simulink model "ame532Project1_GimbalDynamicsModel_2023a_Editing"  (R2023a)
settings: Solver=ode4  StartTime=0.0  StopTime=120  FixedStep=0.01  RelTol=1e-3
model workspace (MAT data in the model file):
  theta = Simulink.Parameter
  theta.DataType = 'auto'
  theta.Complexity = 'real'
  theta.Dimensions = [0 0]
values from neighbouring files (symbols this model uses):
  elevator_sA = 0.435    [Sim_sixDOFdriverScript.m]
  Jxx = 1    [Sim_sixDOFdriverScript.m]
  Jxy = 0.    (= 0)    [Sim_sixDOFdriverScript.m]
  Jxz = 3    [Sim_sixDOFdriverScript.m]
  Jyx = 2    [Sim_sixDOFdriverScript.m]
  Jyy = 2    [Sim_sixDOFdriverScript.m]
  Jyz = 0    [Sim_sixDOFdriverScript.m]
  Jzx = Jxz    (= 3)    [Sim_sixDOFdriverScript.m]
  Jzy = Jyz    (= 0)    [Sim_sixDOFdriverScript.m]
  Jzz = 2    [Sim_sixDOFdriverScript.m]
  leftaileron_sA = 0.192/2    (= 0.096)    [Sim_sixDOFdriverScript.m]
  LL = 0.8    [Sim_sixDOFdriverScript.m]
  MM = 0.8    [Sim_sixDOFdriverScript.m]
  NN = 0.8    [Sim_sixDOFdriverScript.m]
  rEarth = 6378100    [Sim_sixDOFdriverScript.m]
  rightaileron_sA = 0.192/2    (= 0.096)    [Sim_sixDOFdriverScript.m]
  rudder_sA = 0.0333    [Sim_sixDOFdriverScript.m]
  totMass = sum(componentMassesAndGeom(:,1))    [computeMassProps.m]
  x_S2_B_B = (x_S2_B_B_nominal + [0.25*c_s2 0 0]') - x_cg    [computeMassProps.m]
  x_S3_B_B = (x_S3_B_B_nominal + [0.25*c_s3 0 0]') - x_cg    [computeMassProps.m]
  x_S4_B_B = (x_S4_B_B_nominal + [0.25*c_s4 0 0]') - x_cg    [computeMassProps.m]
  x_S5_B_B = (x_S5_B_B_nominal + [0.25*c_s5 0 0]') - x_cg    [computeMassProps.m]
undefined symbols (not defined in the file or in its folder): a0_s2, a0_s3, a0_s4, a0_s5, AR_s2, AR_s3, AR_s4, AR_s5, area_s2, area_s3, area_s4, area_s5, c_s2, c_s3, c_s4, c_s5, CD0_s2, CD0_s3, CD0_s4, CD0_s5, CDa_s2, CDa_s3, CDa_s4, CDa_s5, CL0_s2, CL0_s3, CL0_s4, CL0_s5, CM0_s2, CM0_s3, CM0_s4, CM0_s5, CMa_s2, CMa_s3, CMa_s4, CMa_s5, e_s2, e_s3, e_s4, e_s5, earthRadius, i_s2, i_s3, i_s4, i_s5, n_s2, n_s3, n_s4, n_s5, ro
libraries: simulink_extras x37, matrix_library x26, aerolibutil x6, aerolibfltsims x4, simulink x4, vrlib x3, aerolibtransform2 x2, slpidlib x2, sharedutil x1
(part 1 of 5)
settings Model: Creator=enson  LastModifiedBy=fahee
settings ModelReferenceCC: EnableRefExpFcnMdlSchedulingChecks=on

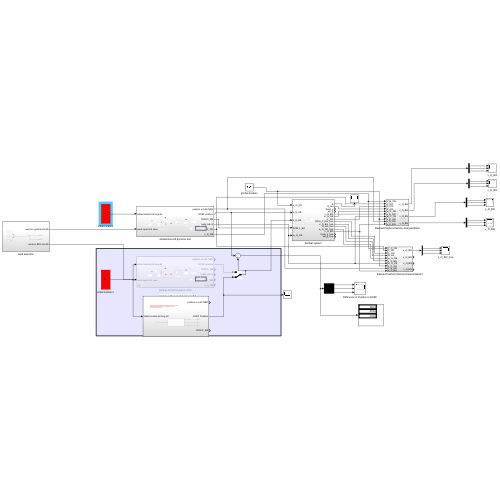
[thumbnail: Simulink's stored preview of the top-level diagram]
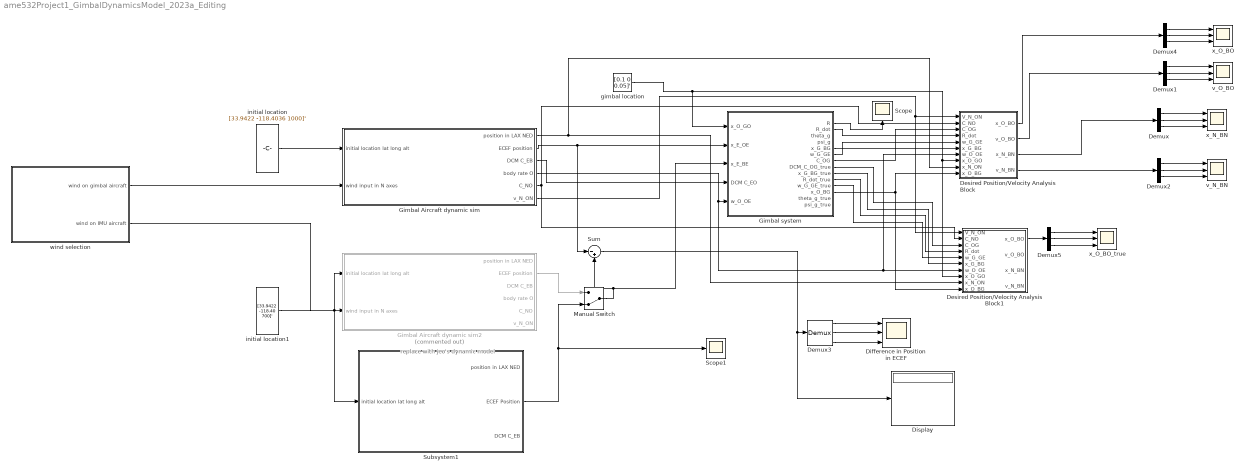
== system ame532Project1_GimbalDynamicsModel_2023a_Editing ==
  note: replace with jeo's dynamic model
  Demux{,1..5} (6 alike) : Demux  Outputs=3
  Desired Position/Velocity Analysis Block : Subsystem
  Desired Position/Velocity Analysis Block1 : Subsystem
  Difference in Position in ECEF : Scope  NumInputPorts=3
  Display : Display
  Gimbal Aircraft dynamic sim : Subsystem
  Gimbal Aircraft dynamic sim2 : Subsystem  Commented=on
  Gimbal system : Subsystem
  Manual Switch : ManualSwitch  CurrentSetting=0
  Scope : Scope
  Scope1 : Scope
  Subsystem1 : Subsystem
  Sum : Sum  Inputs=|-+
  gimbal location : Constant  Value=[0.1 0 0.05]'
  initial location : Constant  Value=[33.9422 -118.4036 1000]'
  initial location1 : Constant  Value=[33.9422 -118.40 700]'
  v_N_BN : Scope  NumInputPorts=3
  v_O_BO : Scope  NumInputPorts=3
  wind selection : Subsystem
  x_N_BN : Scope  NumInputPorts=3
  x_O_BO : Scope  NumInputPorts=3
  x_O_BO_true : Scope  NumInputPorts=3
  wires:
  gimbal location/1 -> Gimbal system/1(x_O_GO), Desired Position/Velocity Analysis Block1/8(x_O_GO), Desired Position/Velocity Analysis Block/8(x_O_GO)
  Gimbal Aircraft dynamic sim/2(ECEF position) -> Sum/1, Gimbal system/2(x_E_OE)
  Manual Switch/1 -> Sum/2, Gimbal system/3(x_E_BE)
  Gimbal system/1(R) -> Scope/1
  Gimbal Aircraft dynamic sim/3(DCM C_EB) -> Gimbal system/4(DCM C_EO)
  Demux3/3 -> Difference in Position in ECEF/3
  Demux3/2 -> Difference in Position in ECEF/2
  Demux3/1 -> Difference in Position in ECEF/1
  Sum/1 -> Display/1, Demux3/1
  initial location/1 -> Gimbal Aircraft dynamic sim/1(initial location lat long alt)
  initial location1/1 -> Subsystem1/1(initial location lat long alt), Gimbal Aircraft dynamic sim2/1(initial location lat long alt)
  Gimbal Aircraft dynamic sim/4(body rate O) -> Desired Position/Velocity Analysis Block/7(w_O_OE), Desired Position/Velocity Analysis Block1/7(w_O_OE), Gimbal system/5(w_O_OE)
  Gimbal system/7(C_OG) -> Desired Position/Velocity Analysis Block/3(C_OG)
  Gimbal system/5(x_G_BG) -> Desired Position/Velocity Analysis Block/6(x_G_BG)
  Gimbal Aircraft dynamic sim/1(position in LAX NED) -> Desired Position/Velocity Analysis Block1/9(x_N_ON), Desired Position/Velocity Analysis Block/9(x_N_ON)
  Gimbal system/2(R_dot) -> Desired Position/Velocity Analysis Block/4(R_dot)
  Gimbal system/6(w_G_GE) -> Desired Position/Velocity Analysis Block/5(w_G_GE)
  Gimbal Aircraft dynamic sim/5(C_NO) -> Desired Position/Velocity Analysis Block1/2(C_NO), Desired Position/Velocity Analysis Block/2(C_NO)
  Gimbal Aircraft dynamic sim/6(v_N_ON) -> Desired Position/Velocity Analysis Block1/1(V_N_ON), Desired Position/Velocity Analysis Block/1(V_N_ON)
  Desired Position/Velocity Analysis Block/3(x_N_BN) -> Demux/1
  Demux/1 -> x_N_BN/1
  Demux/2 -> x_N_BN/2
  Demux/3 -> x_N_BN/3
  Subsystem1/2(ECEF Position) -> Scope1/1, Manual Switch/2
  Gimbal Aircraft dynamic sim2/2(ECEF position) -> Manual Switch/1
  Gimbal system/9(x_G_BG_true) -> Desired Position/Velocity Analysis Block1/6(x_G_BG)
  Gimbal system/11(w_G_GE_true) -> Desired Position/Velocity Analysis Block1/5(w_G_GE)
  Gimbal system/10(R_dot_true) -> Desired Position/Velocity Analysis Block1/4(R_dot)
  Gimbal system/8(DCM_C_OG_true) -> Desired Position/Velocity Analysis Block1/3(C_OG)
  Gimbal system/12(x_O_BG) -> Desired Position/Velocity Analysis Block1/10(x_O_BG), Desired Position/Velocity Analysis Block/10(x_O_BG)
  Desired Position/Velocity Analysis Block/2(v_O_BO) -> Demux1/1
  Demux1/2 -> v_O_BO/2
  Demux1/1 -> v_O_BO/1
  Demux1/3 -> v_O_BO/3
  Desired Position/Velocity Analysis Block/4(v_N_BN) -> Demux2/1
  Demux2/2 -> v_N_BN/2
  Demux2/1 -> v_N_BN/1
  Demux2/3 -> v_N_BN/3
  Desired Position/Velocity Analysis Block/1(x_O_BO) -> Demux4/1
  Demux4/2 -> x_O_BO/2
  Demux4/1 -> x_O_BO/1
  Demux4/3 -> x_O_BO/3
  Desired Position/Velocity Analysis Block1/1(x_O_BO) -> Demux5/1
  Demux5/1 -> x_O_BO_true/1
  Demux5/3 -> x_O_BO_true/3
  Demux5/2 -> x_O_BO_true/2
  wind selection/1(wind on gimbal aircraft) -> Gimbal Aircraft dynamic sim/2(wind input in N axes)
  wind selection/2(wind on IMU aircraft) -> Gimbal Aircraft dynamic sim2/2(wind input in N axes)

== system ame532Project1_GimbalDynamicsModel_2023a_Editing/Desired Position//Velocity Analysis Block ==
  note: position of IMU aircraft w.r.t gimbal + position of gimbal w.r.t gimbal aircraft = position of IMU aircraft w.r.t gimbal aircraft in gimbal coordinates
  note: position of gimbal aircraft w.r.t NED in NED frame
  note: position of gimbal w.r.t aircraft in aircraft frame
  note: position of gimbal aircraft w.r.t Earth in gimbal aircraft frame
  note: Position of IMU aircraft w.r.t the Gimbal in Gimbal Frame
  note: gimbal rates w.r.t Earth in Gimbal frame
  note: derivative of distance from gimbal to IMU aircraft
  note: DCM gimbal to gimbal aircraft
  note: DCM gimbal aircraft to NED
  note: velocity of gimbal aircraft w.r.t NED
  V_N_ON : Inport
  C_NO : Inport  Port=2
  C_OG : Inport  Port=3
  R_dot : Inport  Port=4
  w_G_GE : Inport  Port=5
  x_G_BG : Inport  Port=6
  w_O_OE : Inport  Port=7
  x_O_GO : Inport  Port=8
  x_N_ON : Inport  Port=9
  x_O_BG : Inport  Port=10
  Constant : Constant  Value=0
  Constant1 : Constant  Value=0
  Cross Product : matrix_library/Cross Product
  Cross Product1 : matrix_library/Cross Product
  Display{,1..3,5..6} (6 alike) : Display
  Matrix Multiply{,1..8} (9 alike) : Product  Multiplication=Matrix(*)
  Mux : Mux  Inputs=3
  Scope : Scope
  Scope1 : Scope
  Scope2 : Scope
  Sum : Sum  Inputs=|++
  Sum1 : Sum  Inputs=|++
  Sum2 : Sum  Inputs=|+++
  Sum3 : Sum  Inputs=|++
  Sum4 : Sum  Inputs=|+++
  x_O_BO : Outport
  v_O_BO : Outport  Port=2
  x_N_BN : Outport  Port=3
  v_N_BN : Outport  Port=4
  wires:
  x_O_GO/1 -> Matrix Multiply3/2, Sum/1
  C_OG/1 -> Matrix Multiply5/1, Matrix Multiply2/1, Matrix Multiply1/1, Display5/1, Matrix Multiply/1
  x_G_BG/1 -> Matrix Multiply/2, Matrix Multiply2/2
  Matrix Multiply/1 -> Display3/1, Sum/2
  Sum/1 -> Matrix Multiply7/2, x_O_BO/1
  Constant/1 -> Mux/2
  Constant1/1 -> Mux/3
  R_dot/1 -> Mux/1
  Mux/1 -> Matrix Multiply1/2
  Matrix Multiply1/1 -> Sum3/1, Sum1/1
  Matrix Multiply2/1 -> Cross Product/2
  Cross Product/1 -> Sum1/2, Sum3/2
  Sum1/1 -> v_O_BO/1
  x_N_ON/1 -> Display2/1, Sum2/1, Scope2/1
  C_NO/1 -> Matrix Multiply8/1, Matrix Multiply7/1, Matrix Multiply6/1, Display6/1, Matrix Multiply4/1, Matrix Multiply3/1
  Matrix Multiply3/1 -> Display1/1, Scope/1, Sum2/2
  Matrix Multiply4/1 -> Display/1, Scope1/1, Sum2/3
  Sum2/1 -> x_N_BN/1
  Sum3/1 -> Matrix Multiply6/2
  Matrix Multiply7/1 -> Cross Product1/2
  Matrix Multiply8/1 -> Cross Product1/1
  w_O_OE/1 -> Matrix Multiply8/2
  Cross Product1/1 -> Sum4/3
  Sum4/1 -> v_N_BN/1
  Matrix Multiply6/1 -> Sum4/1
  V_N_ON/1 -> Sum4/2
  x_O_BG/1 -> Matrix Multiply4/2
  w_G_GE/1 -> Matrix Multiply5/2
  Matrix Multiply5/1 -> Cross Product/1

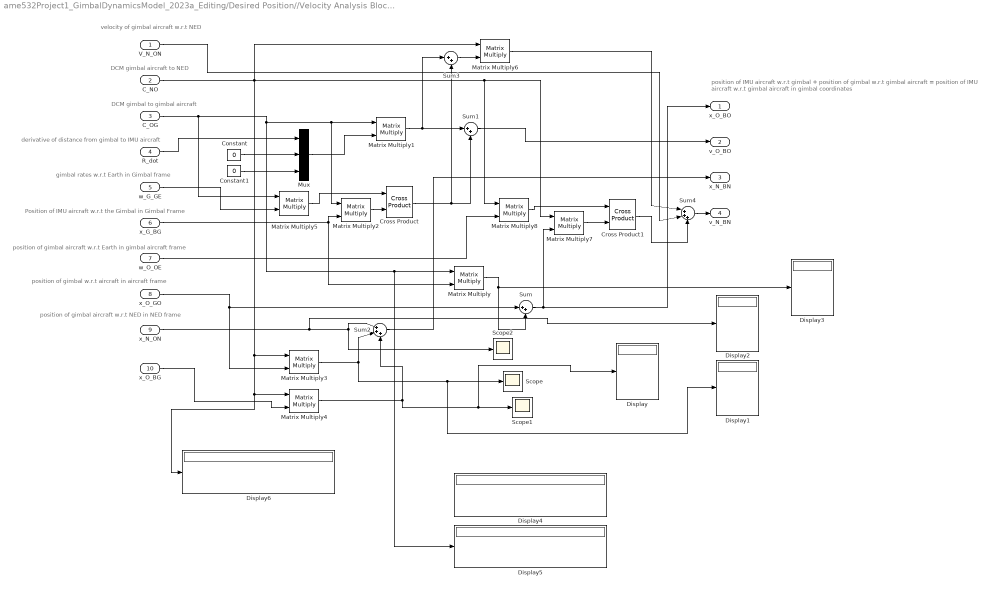
== system ame532Project1_GimbalDynamicsModel_2023a_Editing/Desired Position//Velocity Analysis Block1 ==
  note: position of IMU aircraft w.r.t gimbal + position of gimbal w.r.t gimbal aircraft = position of IMU aircraft w.r.t gimbal aircraft in gimbal coordinates
  note: position of gimbal aircraft w.r.t NED in NED frame
  note: position of gimbal w.r.t aircraft in aircraft frame
  note: position of gimbal aircraft w.r.t Earth in gimbal aircraft frame
  note: Position of IMU aircraft w.r.t the Gimbal in Gimbal Frame
  note: gimbal rates w.r.t Earth in Gimbal frame
  note: derivative of distance from gimbal to IMU aircraft
  note: DCM gimbal to gimbal aircraft
  note: DCM gimbal aircraft to NED
  note: velocity of gimbal aircraft w.r.t NED
  V_N_ON : Inport
  C_NO : Inport  Port=2
  C_OG : Inport  Port=3
  R_dot : Inport  Port=4
  w_G_GE : Inport  Port=5
  x_G_BG : Inport  Port=6
  w_O_OE : Inport  Port=7
  x_O_GO : Inport  Port=8
  x_N_ON : Inport  Port=9
  x_O_BG : Inport  Port=10
  Constant : Constant  Value=0
  Constant1 : Constant  Value=0
  Cross Product : matrix_library/Cross Product
  Cross Product1 : matrix_library/Cross Product
  Display{,1..6} (7 alike) : Display
  Matrix Multiply{,1..8} (9 alike) : Product  Multiplication=Matrix(*)
  Mux : Mux  Inputs=3
  Scope : Scope
  Scope1 : Scope
  Scope2 : Scope
  Sum : Sum  Inputs=|++
  Sum1 : Sum  Inputs=|++
  Sum2 : Sum  Inputs=|+++
  Sum3 : Sum  Inputs=|++
  Sum4 : Sum  Inputs=|+++
  x_O_BO : Outport
  v_O_BO : Outport  Port=2
  x_N_BN : Outport  Port=3
  v_N_BN : Outport  Port=4
  wires:
  x_O_GO/1 -> Matrix Multiply3/2, Sum/1
  C_OG/1 -> Matrix Multiply5/1, Matrix Multiply2/1, Matrix Multiply1/1, Display5/1, Matrix Multiply/1
  x_G_BG/1 -> Matrix Multiply/2, Matrix Multiply2/2
  Matrix Multiply/1 -> Display3/1, Sum/2
  Sum/1 -> Matrix Multiply7/2, x_O_BO/1
  Constant/1 -> Mux/2
  Constant1/1 -> Mux/3
  R_dot/1 -> Mux/1
  Mux/1 -> Matrix Multiply1/2
  Matrix Multiply1/1 -> Sum3/1, Sum1/1
  Matrix Multiply2/1 -> Cross Product/2
  Cross Product/1 -> Sum1/2, Sum3/2
  Sum1/1 -> v_O_BO/1
  x_N_ON/1 -> Display2/1, Sum2/1, Scope2/1
  C_NO/1 -> Matrix Multiply8/1, Matrix Multiply7/1, Matrix Multiply6/1, Display6/1, Matrix Multiply4/1, Matrix Multiply3/1
  Matrix Multiply3/1 -> Display1/1, Scope/1, Sum2/2
  Matrix Multiply4/1 -> Display/1, Scope1/1, Sum2/3
  Sum2/1 -> x_N_BN/1
  Sum3/1 -> Matrix Multiply6/2
  Matrix Multiply7/1 -> Cross Product1/2
  Matrix Multiply8/1 -> Cross Product1/1
  w_O_OE/1 -> Matrix Multiply8/2
  Cross Product1/1 -> Sum4/3
  Sum4/1 -> v_N_BN/1
  Matrix Multiply6/1 -> Sum4/1
  V_N_ON/1 -> Sum4/2
  x_O_BG/1 -> Matrix Multiply4/2
  w_G_GE/1 -> Matrix Multiply5/2
  Matrix Multiply5/1 -> Cross Product/1

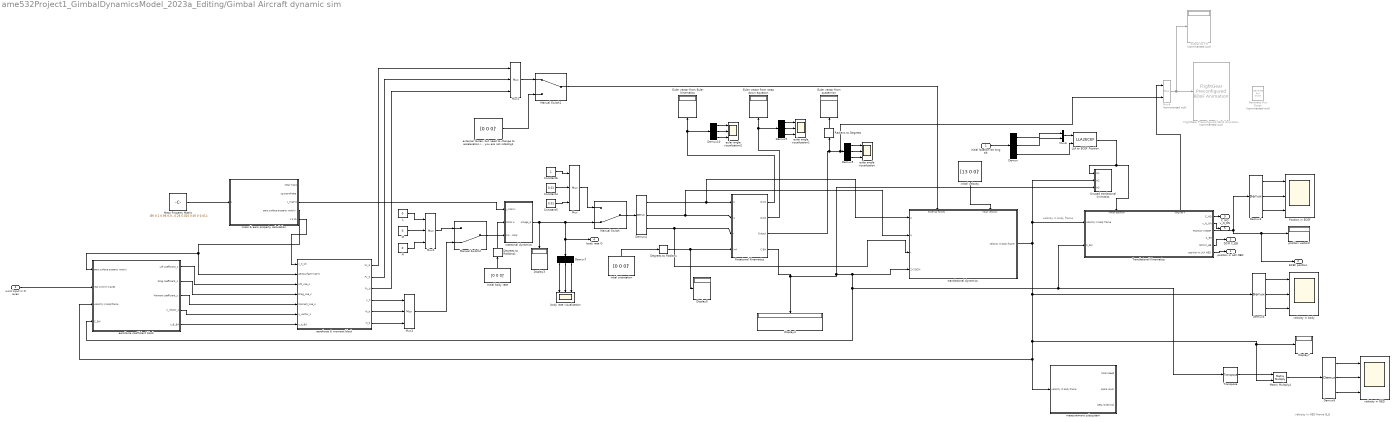
== system ame532Project1_GimbalDynamicsModel_2023a_Editing/Gimbal Aircraft dynamic sim ==
  note: velocity in NED frame B_E
  note: velocity in body frame
  initial location lat long alt : Inport
  wind input in N axes : Inport  Port=2
  Constant4 : Constant  Value=0.01
  Constant5 : Constant  Value=0.01
  Constant6 : Constant
  Degrees to Radians : simulink_extras/Transformations/Degrees to Radians
  Degrees to Radians1 : simulink_extras/Transformations/Degrees to Radians
  Demux{,3..10} (9 alike) : Demux  Outputs=3
  Display{3..5,7} (4 alike) : Display
  Euler vector from Euler Kinematics : Display
  Euler vector from quaternion : Display
  Euler vector from strap down equation : Display
  FlightGear Preconfigured 6DoF Animation : aerolibfltsims/FlightGear Preconfigured 6DoF Animation  Commented=on  xFlightGearVersion=v2019.1  DestinationIpAddress=127.0.0.1  DestinationPort=5502  SampleTime=-1  packetVersion=24
  Generate Run Script : aerolibfltsims/Generate Run Script  Commented=on  Architecture=Win64  dataFlow=Send  GeometryModelName=c172p  AirportId=KSFO  RunwayId=10L  InitialAltitude=7224  InitialHeading=113  OffsetDistance=4.72  OffsetAzimuth=0  InstallScenery=off  DisableShaders=off  OriginAddress=127.0.0.1  DestinationPort=5502  OriginPort=5505  LocalAddress=127.0.0.1  OutputFileName=runfg.bat  FlightGearBaseDirectory=C:\Program Files\FlightGear 2020.3
  Initial body rate : Constant  Value=[0 0 0]'
  L : Constant  Value=0
  LLA to ECEF Position : LLA2ECEF  ptype=Custom  R=earthRadius
  M : Constant  Value=0
  Manual Switch : ManualSwitch  CurrentSetting=0
  Manual Switch1 : ManualSwitch
  Manual Switch2 : ManualSwitch  CurrentSetting=0
  Mass Property Matrix : Constant  Value=|
      | [90 0.1 0.96 0.01 -0.23 0.44 0; 
      |  90 0.1 0.96 0.01 -0.23 -0.44 0; 
      |  13 0.075 0.35 0.002 -0.76 0 -0.16;
      |  0 0.08 0.002 0.18 -0.76 0 -0.09; 
      |  72 0.065 0.035 0.015 -0.05 0 0.03;
      |  106 0.87 0.07 0.07 -0.4 0 0;
      |  27 0.05 0.03 0.005 -0.05 0 0.02; 
      |  10 0.04 0.02 0.005 -0.1 0 0.02;
      |  20 0.05 0.01 0.01 -0.014 0 0; 
      |  40 0.03 0.02 0.02 0.02 0 0.01; 
      |  12 0 0.26 0.025 0.05 0 0.01];
  Matrix Multiply4 : Product  Multiplication=Matrix(*)
  Mux{,1..3} (4 alike) : Mux  Inputs=3
  Mux4 : Mux  Commented=on  Inputs=2
  Mux6 : Mux  Inputs=2
  N : Constant  Value=0
  Position in ECEF : Scope  NumInputPorts=3
  Radians to Degrees : simulink_extras/Transformations/Radians to Degrees
  Rotational Kinematics : Subsystem
  Translational Kinematics : Subsystem
      settings: PortSchema="{\"entries\":[{\"content\":{\"sides\":[{\"content\":{\"connectorIds\":[\"In1\",\"In2\"]},\"type\":\"ConnectorPlacement.EquallySpacedRectSide\",\"uuid\":\"6a5083c9-3149-4656-b001-28ffe3d04409\"},{\"content\":{\"connectorIds\":[\"Out1\",\"Out2\",\"Out3\",\"Out4\",\"Out5\",\"Out6\"],\"side\":\"RIGHT\"},\"type\":\"ConnectorPlacement.EquallySpacedRectSide\",\"uuid\":\"fa51dba7-7f70-4cf9-abef-b6efe75fc937\"},{\"content\":{\"connectorIds\":[\"In3\",\"Out7\"],\"side\":\"TOP\"},\"type\":\"ConnectorPlacement.EquallySpacedRectSide\",\"uuid\":\"76f1511e-a5f6-41ee-949f-b44acacf362b\"}]},\"type\":\"ConnectorPlacement.EquallySpacedConnector\",\"uuid\":\"9a334045-2485-41ee-8c4a-be73d098fd92\"}],\"packageUris\":[\"http://schema.mathworks.com/mf0/Connector/R2020b\"],\"version\":\"1.0\"}"
  Transpose : matrix_library/Transpose
  Unused tranlational kinmatics : Subsystem
  aeroforce & moment block : Subsystem
  aeroforce coefficient block : Subsystem
  body rate visualization : Scope  NumInputPorts=3
  euler angle visualization : Scope  NumInputPorts=3
  euler angle visualization1 : Scope  NumInputPorts=3
  euler angle visualization2 : Scope  NumInputPorts=3
  "external forces, but need to change to acceleration in body these terms should also be corrected with DCM unless you are not rotating1" : Constant  Value=[0 0 0]'
  initial velocity : Constant  Value=[13 0 0]'
  intial orientation : Constant  Value=[0 0 0]'  VectorParams1D=off
  mass & aero property calculation : Subsystem
  measurement subsystem : Subsystem
  output to FG : Display  Commented=on
  position vector3 : Display
  rotational dynamics : Subsystem
  translational dynamics : Subsystem
      settings: PortSchema="{\"entries\":[{\"content\":{\"sides\":[{\"content\":{\"connectorIds\":[\"In1\",\"In2\",\"In3\",\"In4\"]},\"type\":\"ConnectorPlacement.EquallySpacedRectSide\",\"uuid\":\"eb52c09d-c71f-42a1-8e21-86a86e354291\"},{\"content\":{\"connectorIds\":[\"Out1\"],\"side\":\"RIGHT\"},\"type\":\"ConnectorPlacement.EquallySpacedRectSide\",\"uuid\":\"c050fdd0-50ab-42c8-8490-bbe72862ad59\"},{\"content\":{\"connectorIds\":[\"In5\",\"In6\"],\"side\":\"TOP\"},\"type\":\"ConnectorPlacement.EquallySpacedRectSide\",\"uuid\":\"d308cee2-bf9d-4ab9-b003-c94f4b2955f2\"},{\"content\":{\"connectorIds\":[],\"side\":\"BOTTOM\"},\"type\":\"ConnectorPlacement.EquallySpacedRectSide\",\"uuid\":\"cf51bcec-71dd-45f1-b1ae-be572a1ab1ac\"}]},\"type\":\"ConnectorPlacement.EquallySpacedConnector\",\"uuid\":\"72e461db-b4a1-4e87-8f9d-278a55fe116d\"}],\"packageUris\":[\"http://schema.mathworks.com/mf0/Connector/R2020b\"],\"version\":\"1.0\"}"
  velocity in NED : Scope  NumInputPorts=3
  velocity in body : Scope  NumInputPorts=3
  position in LAX NED : Outport
  ECEF position : Outport  Port=2
  DCM C_EB : Outport  Port=3
  body rate O : Outport  Port=4
  C_NO : Outport  Port=5
  v_N_ON : Outport  Port=6
  wires:
  translational dynamics/1(velocity in body frame) -> measurement subsystem/1(velocity in body frame), aeroforce coefficient block/3(velocity in bodyframe), Matrix Multiply4/2, Display7/1, Demux6/1, Translational Kinematics/1(velocity in body frame), Unused tranlational kinmatics/2(In2)
  Translational Kinematics/3(Position in ECEF) -> Demux3/1, ECEF position/1, position vector3/1
  aeroforce coefficient block/4(n_vector_s) -> aeroforce & moment block/6(n_vector_s)
  aeroforce & moment block/1(Fx_b) -> Mux1/1
  Demux3/2 -> Position in ECEF/2
  Demux6/3 -> velocity in body/3
  Demux4/3 -> translational dynamics/3(r), Rotational Kinematics/3(r)
  L/1 -> Mux2/1
  Initial body rate/1 -> Degrees to Radians1/1
  mass & aero property calculation/4(aero surface property matrix) -> aeroforce & moment block/2(aerosurface matrix), aeroforce coefficient block/1(aero surface property matrix)
  Rotational Kinematics/1(Out1) -> Demux10/1, Euler vector from Euler Kinematics/1
  aeroforce & moment block/5(M_b) -> Mux3/2
  Demux4/2 -> Rotational Kinematics/2(q), translational dynamics/2(q)
  LLA to ECEF Position/1 -> Unused tranlational kinmatics/1(In1), Translational Kinematics/3(initial position)
  Rotational Kinematics/2(Out2) -> Euler vector from strap down equation/1, Demux9/1
  intial orientation/1 -> Degrees to Radians/1
  aeroforce & moment block/3(Fz_b) -> Mux1/3
  aeroforce coefficient block/3(Moment coefficient_s) -> aeroforce & moment block/5(Moment_coe_s)
  Rotational Kinematics/4(C BN) -> Display4/1, Unused tranlational kinmatics/3(In3), Transpose/1, Translational Kinematics/2(C_BN), aeroforce coefficient block/4(C_BN), translational dynamics/4(ZYXDCM)
  Manual Switch1/1 -> translational dynamics/5(external forces)
  Rotational Kinematics/3(Output) -> Mux4/2, Demux5/1, Radians to Degrees/1
  wind input in N axes/1 -> aeroforce coefficient block/2(real wind in N axes)
  initial velocity/1 -> translational dynamics/6(intial velocity)
  Mass Property Matrix/1 -> mass & aero property calculation/1(u)
  Constant4/1 -> Mux/2
  Mux2/1 -> Manual Switch2/1
  Demux9/2 -> euler angle visualization1/2
  rotational dynamics/1(omega_b) -> Manual Switch/2, body rate O/1, Demux7/1, Display3/1
  Degrees to Radians/1 -> Display5/1, Rotational Kinematics/4(In4)
  Demux6/2 -> velocity in body/2
  Demux5/3 -> euler angle visualization/3
  aeroforce coefficient block/1(Lift coefficient_s) -> aeroforce & moment block/3(Lift_coe_s)
  Mux/1 -> Manual Switch/1
  Demux7/1 -> body rate visualization/1
  Constant5/1 -> Mux/3
  mass & aero property calculation/5(x b sb) -> aeroforce & moment block/1(x_b_sb)
  Demux7/3 -> body rate visualization/3
  Transpose/1 -> Matrix Multiply4/1
  "external forces, but need to change to acceleration in body these terms should also be corrected with DCM unless you are not rotating1"/1 -> Manual Switch1/2
  Mux4/1 -> output to FG/1, FlightGear Preconfigured 6DoF Animation/1
  Constant6/1 -> Mux/1
  aeroforce & moment block/2(Fy_b) -> Mux1/2
  aeroforce coefficient block/5(v_B_BA) -> aeroforce & moment block/7(v_b_BA)
  N/1 -> Mux2/3
  Demux7/2 -> body rate visualization/2
  aeroforce & moment block/4(L_b) -> Mux3/1
  Demux8/2 -> velocity in NED/2
  Demux9/3 -> euler angle visualization1/3
  aeroforce & moment block/6(N_b) -> Mux3/3
  Demux4/1 -> translational dynamics/1(p), Rotational Kinematics/1(p)
  Demux10/2 -> euler angle visualization2/2
  Mux3/1 -> Manual Switch2/2
  mass & aero property calculation/3(J_matrix) -> rotational dynamics/1(J_matrix)
  Demux10/3 -> euler angle visualization2/3
  aeroforce coefficient block/2(Drag coefficient_s) -> aeroforce & moment block/4(Drag_coe_s)
  Demux10/1 -> euler angle visualization2/1
  Manual Switch/1 -> Demux4/1
  Translational Kinematics/7(long lat h) -> Mux4/1
  Demux3/3 -> Position in ECEF/3
  Demux8/1 -> velocity in NED/1
  Demux5/2 -> euler angle visualization/2
  Mux1/1 -> Manual Switch1/1
  Manual Switch2/1 -> rotational dynamics/3(moment in body)
  Demux5/1 -> euler angle visualization/1
  M/1 -> Mux2/2
  Demux3/1 -> Position in ECEF/1
  Matrix Multiply4/1 -> Demux8/1
  Radians to Degrees/1 -> Euler vector from quaternion/1
  Demux8/3 -> velocity in NED/3
  Demux9/1 -> euler angle visualization1/1
  Degrees to Radians1/1 -> rotational dynamics/2(Initial w)
  Demux6/1 -> velocity in body/1
  Translational Kinematics/6(position in LAX NED) -> position in LAX NED/1
  Mux6/1 -> LLA to ECEF Position/1
  Translational Kinematics/5(DCM C_EB) -> DCM C_EB/1
  initial location lat long alt/1 -> Demux/1
  Demux/1 -> Mux6/1
  Demux/2 -> Mux6/2
  Demux/3 -> LLA to ECEF Position/2
  Translational Kinematics/1(C_NO) -> C_NO/1
  Translational Kinematics/2(v_N_ON) -> v_N_ON/1

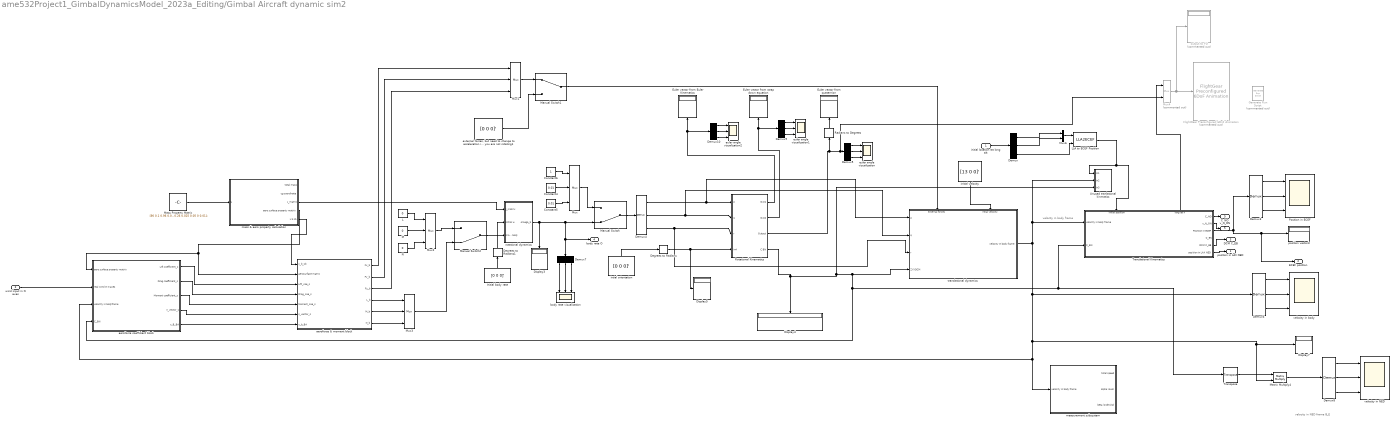
== system ame532Project1_GimbalDynamicsModel_2023a_Editing/Gimbal Aircraft dynamic sim2 ==
  note: velocity in NED frame B_E
  note: velocity in body frame
  initial location lat long alt : Inport
  wind input in N axes : Inport  Port=2
  Constant4 : Constant  Value=0.01
  Constant5 : Constant  Value=0.01
  Constant6 : Constant
  Degrees to Radians : simulink_extras/Transformations/Degrees to Radians
  Degrees to Radians1 : simulink_extras/Transformations/Degrees to Radians
  Demux{,3..10} (9 alike) : Demux  Outputs=3
  Display{3..5,7} (4 alike) : Display
  Euler vector from Euler Kinematics : Display
  Euler vector from quaternion : Display
  Euler vector from strap down equation : Display
  FlightGear Preconfigured 6DoF Animation : aerolibfltsims/FlightGear Preconfigured 6DoF Animation  Commented=on  xFlightGearVersion=v2019.1  DestinationIpAddress=127.0.0.1  DestinationPort=5502  SampleTime=-1  packetVersion=24
  Generate Run Script : aerolibfltsims/Generate Run Script  Commented=on  Architecture=Win64  dataFlow=Send  GeometryModelName=c172p  AirportId=KSFO  RunwayId=10L  InitialAltitude=7224  InitialHeading=113  OffsetDistance=4.72  OffsetAzimuth=0  InstallScenery=off  DisableShaders=off  OriginAddress=127.0.0.1  DestinationPort=5502  OriginPort=5505  LocalAddress=127.0.0.1  OutputFileName=runfg.bat  FlightGearBaseDirectory=C:\Program Files\FlightGear 2020.3
  Initial body rate : Constant  Value=[0 0 0]'
  L : Constant  Value=0
  LLA to ECEF Position : LLA2ECEF  ptype=Custom  R=earthRadius
  M : Constant  Value=0
  Manual Switch : ManualSwitch  CurrentSetting=0
  Manual Switch1 : ManualSwitch
  Manual Switch2 : ManualSwitch  CurrentSetting=0
  Mass Property Matrix : Constant  Value=|
      | [90 0.1 0.96 0.01 -0.23 0.44 0; 
      |  90 0.1 0.96 0.01 -0.23 -0.44 0; 
      |  13 0.075 0.35 0.002 -0.76 0 -0.16;
      |  0 0.08 0.002 0.18 -0.76 0 -0.09; 
      |  72 0.065 0.035 0.015 -0.05 0 0.03;
      |  106 0.87 0.07 0.07 -0.4 0 0;
      |  27 0.05 0.03 0.005 -0.05 0 0.02; 
      |  10 0.04 0.02 0.005 -0.1 0 0.02;
      |  20 0.05 0.01 0.01 -0.014 0 0; 
      |  40 0.03 0.02 0.02 0.02 0 0.01; 
      |  12 0 0.26 0.025 0.05 0 0.01];
  Matrix Multiply4 : Product  Multiplication=Matrix(*)
  Mux{,1..3} (4 alike) : Mux  Inputs=3
  Mux4 : Mux  Commented=on  Inputs=2
  Mux6 : Mux  Inputs=2
  N : Constant  Value=0
  Position in ECEF : Scope  NumInputPorts=3
  Radians to Degrees : simulink_extras/Transformations/Radians to Degrees
  Rotational Kinematics : Subsystem
  Translational Kinematics : Subsystem
      settings: PortSchema="{\"entries\":[{\"content\":{\"sides\":[{\"content\":{\"connectorIds\":[\"In1\",\"In2\"]},\"type\":\"ConnectorPlacement.EquallySpacedRectSide\",\"uuid\":\"6a5083c9-3149-4656-b001-28ffe3d04409\"},{\"content\":{\"connectorIds\":[\"Out1\",\"Out2\",\"Out3\",\"Out4\",\"Out5\",\"Out6\"],\"side\":\"RIGHT\"},\"type\":\"ConnectorPlacement.EquallySpacedRectSide\",\"uuid\":\"fa51dba7-7f70-4cf9-abef-b6efe75fc937\"},{\"content\":{\"connectorIds\":[\"In3\",\"Out7\"],\"side\":\"TOP\"},\"type\":\"ConnectorPlacement.EquallySpacedRectSide\",\"uuid\":\"76f1511e-a5f6-41ee-949f-b44acacf362b\"}]},\"type\":\"ConnectorPlacement.EquallySpacedConnector\",\"uuid\":\"9a334045-2485-41ee-8c4a-be73d098fd92\"}],\"packageUris\":[\"http://schema.mathworks.com/mf0/Connector/R2020b\"],\"version\":\"1.0\"}"
  Transpose : matrix_library/Transpose
  Unused tranlational kinmatics : Subsystem
  aeroforce & moment block : Subsystem
  aeroforce coefficient block : Subsystem
  body rate visualization : Scope  NumInputPorts=3
  euler angle visualization : Scope  NumInputPorts=3
  euler angle visualization1 : Scope  NumInputPorts=3
  euler angle visualization2 : Scope  NumInputPorts=3
  "external forces, but need to change to acceleration in body these terms should also be corrected with DCM unless you are not rotating1" : Constant  Value=[0 0 0]'
  initial velocity : Constant  Value=[13 0 0]'
  intial orientation : Constant  Value=[0 0 0]'  VectorParams1D=off
  mass & aero property calculation : Subsystem
  measurement subsystem : Subsystem
  output to FG : Display  Commented=on
  position vector3 : Display
  rotational dynamics : Subsystem
  translational dynamics : Subsystem
      settings: PortSchema="{\"entries\":[{\"content\":{\"sides\":[{\"content\":{\"connectorIds\":[\"In1\",\"In2\",\"In3\",\"In4\"]},\"type\":\"ConnectorPlacement.EquallySpacedRectSide\",\"uuid\":\"eb52c09d-c71f-42a1-8e21-86a86e354291\"},{\"content\":{\"connectorIds\":[\"Out1\"],\"side\":\"RIGHT\"},\"type\":\"ConnectorPlacement.EquallySpacedRectSide\",\"uuid\":\"c050fdd0-50ab-42c8-8490-bbe72862ad59\"},{\"content\":{\"connectorIds\":[\"In5\",\"In6\"],\"side\":\"TOP\"},\"type\":\"ConnectorPlacement.EquallySpacedRectSide\",\"uuid\":\"d308cee2-bf9d-4ab9-b003-c94f4b2955f2\"},{\"content\":{\"connectorIds\":[],\"side\":\"BOTTOM\"},\"type\":\"ConnectorPlacement.EquallySpacedRectSide\",\"uuid\":\"cf51bcec-71dd-45f1-b1ae-be572a1ab1ac\"}]},\"type\":\"ConnectorPlacement.EquallySpacedConnector\",\"uuid\":\"72e461db-b4a1-4e87-8f9d-278a55fe116d\"}],\"packageUris\":[\"http://schema.mathworks.com/mf0/Connector/R2020b\"],\"version\":\"1.0\"}"
  velocity in NED : Scope  NumInputPorts=3
  velocity in body : Scope  NumInputPorts=3
  position in LAX NED : Outport
  ECEF position : Outport  Port=2
  DCM C_EB : Outport  Port=3
  body rate O : Outport  Port=4
  C_NO : Outport  Port=5
  v_N_ON : Outport  Port=6
  wires:
  translational dynamics/1(velocity in body frame) -> measurement subsystem/1(velocity in body frame), aeroforce coefficient block/3(velocity in bodyframe), Matrix Multiply4/2, Display7/1, Demux6/1, Translational Kinematics/1(velocity in body frame), Unused tranlational kinmatics/2(In2)
  Translational Kinematics/3(Position in ECEF) -> Demux3/1, ECEF position/1, position vector3/1
  aeroforce coefficient block/4(n_vector_s) -> aeroforce & moment block/6(n_vector_s)
  aeroforce & moment block/1(Fx_b) -> Mux1/1
  Demux3/2 -> Position in ECEF/2
  Demux6/3 -> velocity in body/3
  Demux4/3 -> translational dynamics/3(r), Rotational Kinematics/3(r)
  L/1 -> Mux2/1
  Initial body rate/1 -> Degrees to Radians1/1
  mass & aero property calculation/4(aero surface property matrix) -> aeroforce & moment block/2(aerosurface matrix), aeroforce coefficient block/1(aero surface property matrix)
  Rotational Kinematics/1(Out1) -> Demux10/1, Euler vector from Euler Kinematics/1
  aeroforce & moment block/5(M_b) -> Mux3/2
  Demux4/2 -> Rotational Kinematics/2(q), translational dynamics/2(q)
  LLA to ECEF Position/1 -> Unused tranlational kinmatics/1(In1), Translational Kinematics/3(initial position)
  Rotational Kinematics/2(Out2) -> Euler vector from strap down equation/1, Demux9/1
  intial orientation/1 -> Degrees to Radians/1
  aeroforce & moment block/3(Fz_b) -> Mux1/3
  aeroforce coefficient block/3(Moment coefficient_s) -> aeroforce & moment block/5(Moment_coe_s)
  Rotational Kinematics/4(C BN) -> Display4/1, Unused tranlational kinmatics/3(In3), Transpose/1, Translational Kinematics/2(C_BN), aeroforce coefficient block/4(C_BN), translational dynamics/4(ZYXDCM)
  Manual Switch1/1 -> translational dynamics/5(external forces)
  Rotational Kinematics/3(Output) -> Mux4/2, Demux5/1, Radians to Degrees/1
  wind input in N axes/1 -> aeroforce coefficient block/2(real wind in N axes)
  initial velocity/1 -> translational dynamics/6(intial velocity)
  Mass Property Matrix/1 -> mass & aero property calculation/1(u)
  Constant4/1 -> Mux/2
  Mux2/1 -> Manual Switch2/1
  Demux9/2 -> euler angle visualization1/2
  rotational dynamics/1(omega_b) -> Manual Switch/2, body rate O/1, Demux7/1, Display3/1
  Degrees to Radians/1 -> Display5/1, Rotational Kinematics/4(In4)
  Demux6/2 -> velocity in body/2
  Demux5/3 -> euler angle visualization/3
  aeroforce coefficient block/1(Lift coefficient_s) -> aeroforce & moment block/3(Lift_coe_s)
  Mux/1 -> Manual Switch/1
  Demux7/1 -> body rate visualization/1
  Constant5/1 -> Mux/3
  mass & aero property calculation/5(x b sb) -> aeroforce & moment block/1(x_b_sb)
  Demux7/3 -> body rate visualization/3
  Transpose/1 -> Matrix Multiply4/1
  "external forces, but need to change to acceleration in body these terms should also be corrected with DCM unless you are not rotating1"/1 -> Manual Switch1/2
  Mux4/1 -> output to FG/1, FlightGear Preconfigured 6DoF Animation/1
  Constant6/1 -> Mux/1
  aeroforce & moment block/2(Fy_b) -> Mux1/2
  aeroforce coefficient block/5(v_B_BA) -> aeroforce & moment block/7(v_b_BA)
  N/1 -> Mux2/3
  Demux7/2 -> body rate visualization/2
  aeroforce & moment block/4(L_b) -> Mux3/1
  Demux8/2 -> velocity in NED/2
  Demux9/3 -> euler angle visualization1/3
  aeroforce & moment block/6(N_b) -> Mux3/3
  Demux4/1 -> translational dynamics/1(p), Rotational Kinematics/1(p)
  Demux10/2 -> euler angle visualization2/2
  Mux3/1 -> Manual Switch2/2
  mass & aero property calculation/3(J_matrix) -> rotational dynamics/1(J_matrix)
  Demux10/3 -> euler angle visualization2/3
  aeroforce coefficient block/2(Drag coefficient_s) -> aeroforce & moment block/4(Drag_coe_s)
  Demux10/1 -> euler angle visualization2/1
  Manual Switch/1 -> Demux4/1
  Translational Kinematics/7(long lat h) -> Mux4/1
  Demux3/3 -> Position in ECEF/3
  Demux8/1 -> velocity in NED/1
  Demux5/2 -> euler angle visualization/2
  Mux1/1 -> Manual Switch1/1
  Manual Switch2/1 -> rotational dynamics/3(moment in body)
  Demux5/1 -> euler angle visualization/1
  M/1 -> Mux2/2
  Demux3/1 -> Position in ECEF/1
  Matrix Multiply4/1 -> Demux8/1
  Radians to Degrees/1 -> Euler vector from quaternion/1
  Demux8/3 -> velocity in NED/3
  Demux9/1 -> euler angle visualization1/1
  Degrees to Radians1/1 -> rotational dynamics/2(Initial w)
  Demux6/1 -> velocity in body/1
  Translational Kinematics/6(position in LAX NED) -> position in LAX NED/1
  Mux6/1 -> LLA to ECEF Position/1
  Translational Kinematics/5(DCM C_EB) -> DCM C_EB/1
  initial location lat long alt/1 -> Demux/1
  Demux/1 -> Mux6/1
  Demux/2 -> Mux6/2
  Demux/3 -> LLA to ECEF Position/2
  Translational Kinematics/1(C_NO) -> C_NO/1
  Translational Kinematics/2(v_N_ON) -> v_N_ON/1

== system ame532Project1_GimbalDynamicsModel_2023a_Editing/Gimbal system ==
  note: GIMBAL DYNAMICS
  note: GIMBAL KINEMATICS
  note: DISCRETIZED SYSTEM
  note: Radar/Gimbal Measurement
  note: Gimbal Controller
  x_O_GO : Inport
  x_E_OE : Inport  Port=2
  x_E_BE : Inport  Port=3
  DCM C_EO : Inport  Port=4
  w_O_OE : Inport  Port=5
  "Controller " : Subsystem
  Discretized System : Subsystem
  Gimbal Dynamics Model : Subsystem
  Gimbal Kinematics Model : Subsystem
  J_gimbal : Constant  Value=[0.01 0 0; 0 0.01 0; 0 0 0.01]
  Subsystem : Subsystem
  gimbal orientation initial : Constant  Value=[0 0 0]
  w_gimbal_initial : Constant  Value=[0 0 0]
  R : Outport
  R_dot : Outport  Port=2
  theta_g : Outport  Port=3
  psi_g : Outport  Port=4
  x_G_BG : Outport  Port=5
  w_G_GE : Outport  Port=6
  C_OG : Outport  Port=7
  DCM_C_OG_true : Outport  Port=8
  x_G_BG_true : Outport  Port=9
  R_dot_true : Outport  Port=10
  w_G_GE_true : Outport  Port=11
  x_O_BG : Outport  Port=12
  theta_g_true : Outport  Port=13
  psi_g_true : Outport  Port=14
  wires:
  w_gimbal_initial/1 -> Gimbal Dynamics Model/2(Initial w)
  J_gimbal/1 -> Gimbal Dynamics Model/1(J_matrix)
  Gimbal Dynamics Model/1(w_b) -> Gimbal Kinematics Model/3(w_b_dynamics)
  w_O_OE/1 -> Gimbal Kinematics Model/1(w_O_OE), Subsystem/1(In1)
  "Controller "/1(Torque_Cmd) -> Gimbal Dynamics Model/3(Tcmd)
  Gimbal Kinematics Model/3(psi_g_true) -> Discretized System/4(psi_g_true), psi_g_true/1
  Gimbal Kinematics Model/1(C_OG_true) -> DCM_C_OG_true/1
  Gimbal Kinematics Model/2(theta_g_true) -> Discretized System/2(theta_g_true), theta_g_true/1
  gimbal orientation initial/1 -> Gimbal Kinematics Model/4(eul_GO_0)
  Gimbal Kinematics Model/4(w_G_GE_true) -> w_G_GE_true/1
  Gimbal Kinematics Model/5(eul_GO_Deg) -> "Controller "/2(GA_True)
  Discretized System/1(Out1) -> x_G_BG_true/1
  Discretized System/2(Out2) -> R_dot_true/1
  DCM C_EO/1 -> Subsystem/2(In2)
  x_O_GO/1 -> Subsystem/3(In3)
  x_E_OE/1 -> Subsystem/4(In4)
  x_E_BE/1 -> Subsystem/5(In5)
  Subsystem/1(C_OG) -> C_OG/1
  Subsystem/2(w_G_GE) -> w_G_GE/1
  Subsystem/3(theta in degrees) -> theta_g/1
  Subsystem/6(x_O_BG) -> x_O_BG/1
  Subsystem/7(w_G_GO) -> Gimbal Kinematics Model/2(w_b_measurement)
  Subsystem/5(psi in degree) -> psi_g/1, Discretized System/3(psi_g_measured)
  Subsystem/8(Gimbal Euler Angles) -> "Controller "/1(GA_Desired)
  Subsystem/9(R) -> R/1
  Subsystem/4(theta in radian) -> Discretized System/1(theta_g_measured)
  Subsystem/10(R_dot) -> Discretized System/5(Rdot), R_dot/1
  Subsystem/11(x_G_BG) -> Discretized System/6(x_G_BG), x_G_BG/1

== system ame532Project1_GimbalDynamicsModel_2023a_Editing/Subsystem1 ==
  note: NOTE: RUN "Sim_sixDOFdriverScript.m" script first as it initializes model parameters and workspace for the simulink model to access
  initial location lat long alt : Inport
  Equations of Motion : Subsystem
  position in LAX NED : Outport
  ECEF Position : Outport  Port=2
  DCM C_EB : Outport  Port=3
  wires:
  initial location lat long alt/1 -> Equations of Motion/1(initial location lat long alt)
  Equations of Motion/2(position in LAX NED) -> position in LAX NED/1
  Equations of Motion/1(Out Positon E_x_B_E_E) -> ECEF Position/1
  Equations of Motion/3(DCM C_EB) -> DCM C_EB/1

== system ame532Project1_GimbalDynamicsModel_2023a_Editing/wind selection ==
  Mux : Mux  Inputs=3
  V_Wind_X : Step  Time=0  After=0  SampleTime=0
  V_Wind_Y : Step  Time=0  After=0  SampleTime=0
  V_Wind_Z : Step  Time=0  After=0  SampleTime=0
  wind on gimbal aircraft : Outport
  wind on IMU aircraft : Outport  Port=2
  wires:
  V_Wind_X/1 -> Mux/1
  V_Wind_Y/1 -> Mux/2
  V_Wind_Z/1 -> Mux/3
  Mux/1 -> wind on IMU aircraft/1, wind on gimbal aircraft/1

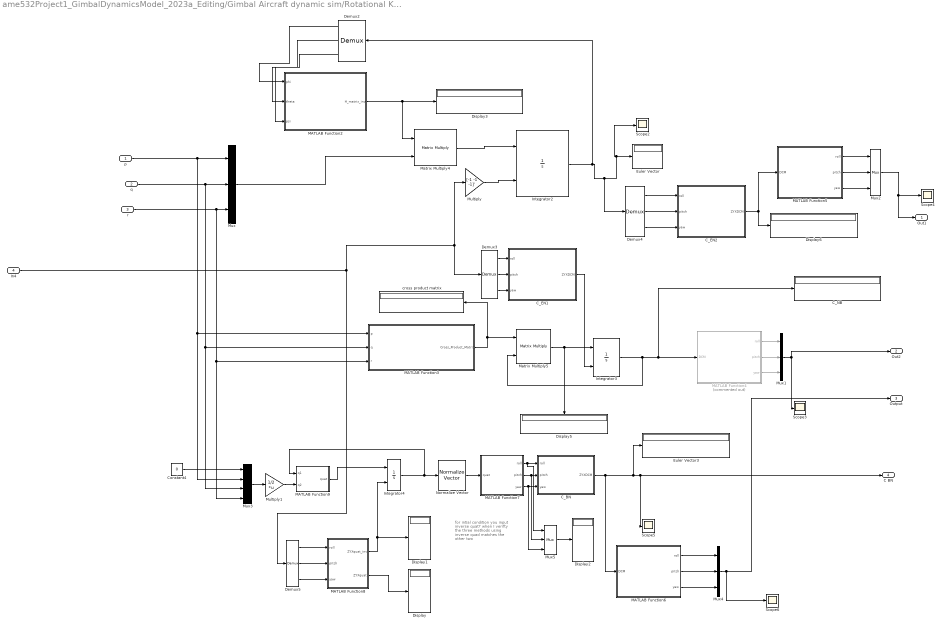
== system ame532Project1_GimbalDynamicsModel_2023a_Editing/Gimbal Aircraft dynamic sim/Rotational Kinematics ==
  note: for intial condition you input inverse quat?
      | when I verifty the three methods using inverse quad matches the other two
  p : Inport
  q : Inport  Port=2
  r : Inport  Port=3
  In4 : Inport  Port=4
  C_BN : MATLAB Function  TreatAsAtomicUnit=on
  C_EN1 : MATLAB Function  TreatAsAtomicUnit=on
  C_EN2 : MATLAB Function  TreatAsAtomicUnit=on
  C_NB : Display
  Constant4 : Constant  Value=0
  Demux{2..5} (4 alike) : Demux  Outputs=3
  Display{,1..3,5..6} (6 alike) : Display
  Euler Vector : Display
  Euler Vector3 : Display
  Integrator2 : Integrator  InitialConditionSource=external
  Integrator3 : Integrator  InitialConditionSource=external
  Integrator4 : Integrator  InitialConditionSource=external  InitialCondition=[1 0 0 0]'
  MATLAB Function2 : MATLAB Function  TreatAsAtomicUnit=on
  MATLAB Function3 : MATLAB Function  TreatAsAtomicUnit=on
  MATLAB Function4 : MATLAB Function  Commented=on  TreatAsAtomicUnit=on
  MATLAB Function5 : MATLAB Function  TreatAsAtomicUnit=on
  MATLAB Function6 : MATLAB Function  TreatAsAtomicUnit=on
  MATLAB Function7 : MATLAB Function  TreatAsAtomicUnit=on
  MATLAB Function8 : MATLAB Function  TreatAsAtomicUnit=on
  MATLAB Function9 : MATLAB Function  TreatAsAtomicUnit=on
  Matrix Multiply4 : Product  Multiplication=Matrix(*)
  Matrix Multiply5 : Product  Multiplication=Matrix(*)
  Multiply : Gain  Gain=[-1 -1 -1]'
  Multiply1 : Gain  Gain=1/2  Multiplication=Matrix(K*u)
  Mux{,1..2,4..5} (5 alike) : Mux  Inputs=3
  Mux3 : Mux
  Normalize Vector : vrlib/Utilities/Normalize Vector  maxzero=0
  Scope{2..6} (5 alike) : Scope
  cross product matrix : Display
  Out1 : Outport
  Out2 : Outport  Port=2
  Output : Outport  Port=3
  C BN : Outport  Port=4
  wires:
  Matrix Multiply4/1 -> Integrator2/1
  In4/1 -> Multiply/1, Demux3/1, Demux5/1
  MATLAB Function4/3(yaw) -> Mux1/3
  Integrator2/1 -> Scope2/1, Euler Vector/1, Demux4/1, Demux2/1
  MATLAB Function2/1(H_matrix_inv) -> Display3/1, Matrix Multiply4/1
  MATLAB Function6/2(pitch) -> Mux4/2
  r/1 -> Mux3/4, MATLAB Function3/3(r), Mux/3
  Matrix Multiply5/1 -> Display5/1, Integrator3/1
  Mux/1 -> Matrix Multiply4/2
  q/1 -> Mux3/3, MATLAB Function3/2(q), Mux/2
  C_BN/1(ZYXDCM) -> MATLAB Function6/1(DCM), C BN/1, Scope5/1, Euler Vector3/1
  C_EN1/1(ZYXDCM) -> Integrator3/2
  MATLAB Function5/2(pitch) -> Mux2/2
  Mux1/1 -> Out2/1, Scope3/1
  MATLAB Function4/1(roll) -> Mux1/1
  Demux2/2 -> MATLAB Function2/2(theta)
  Demux4/3 -> C_EN2/3(yaw)
  MATLAB Function4/2(pitch) -> Mux1/2
  Demux2/3 -> MATLAB Function2/3(psi)
  Demux2/1 -> MATLAB Function2/1(phi)
  Demux5/1 -> MATLAB Function8/1(roll)
  Demux3/1 -> C_EN1/1(roll)
  Demux5/2 -> MATLAB Function8/2(pitch)
  Demux4/1 -> C_EN2/1(roll)
  Demux3/3 -> C_EN1/3(yaw)
  Multiply/1 -> Integrator2/2
  C_EN2/1(ZYXDCM) -> Display6/1, MATLAB Function5/1(DCM)
  Normalize Vector/1 -> MATLAB Function7/1(quat)
  MATLAB Function9/1(quat) -> Integrator4/1
  Integrator3/1 -> Matrix Multiply5/2, MATLAB Function4/1(DCM), C_NB/1
  p/1 -> Mux3/2, MATLAB Function3/1(p), Mux/1
  Integrator4/1 -> Normalize Vector/1, MATLAB Function9/1(q1)
  MATLAB Function7/3(yaw) -> Mux5/3, C_BN/3(yaw)
  Mux2/1 -> Out1/1, Scope4/1
  MATLAB Function5/3(yaw) -> Mux2/3
  Constant4/1 -> Mux3/1
  Mux3/1 -> Multiply1/1
  Mux4/1 -> Output/1, Scope6/1
  MATLAB Function7/1(roll) -> Mux5/1, C_BN/1(roll)
  MATLAB Function5/1(roll) -> Mux2/1
  Demux5/3 -> MATLAB Function8/3(yaw)
  MATLAB Function6/1(roll) -> Mux4/1
  MATLAB Function6/3(yaw) -> Mux4/3
  Multiply1/1 -> MATLAB Function9/2(q2)
  MATLAB Function3/1(Cross_Product_Matrix) -> Matrix Multiply5/1, cross product matrix/1
  Demux4/2 -> C_EN2/2(pitch)
  Demux3/2 -> C_EN1/2(pitch)
  MATLAB Function7/2(pitch) -> Mux5/2, C_BN/2(pitch)
  MATLAB Function8/1(ZYXquat_inv) -> Integrator4/2, Display1/1
  MATLAB Function8/2(ZYXquat) -> Display/1
  Mux5/1 -> Display2/1

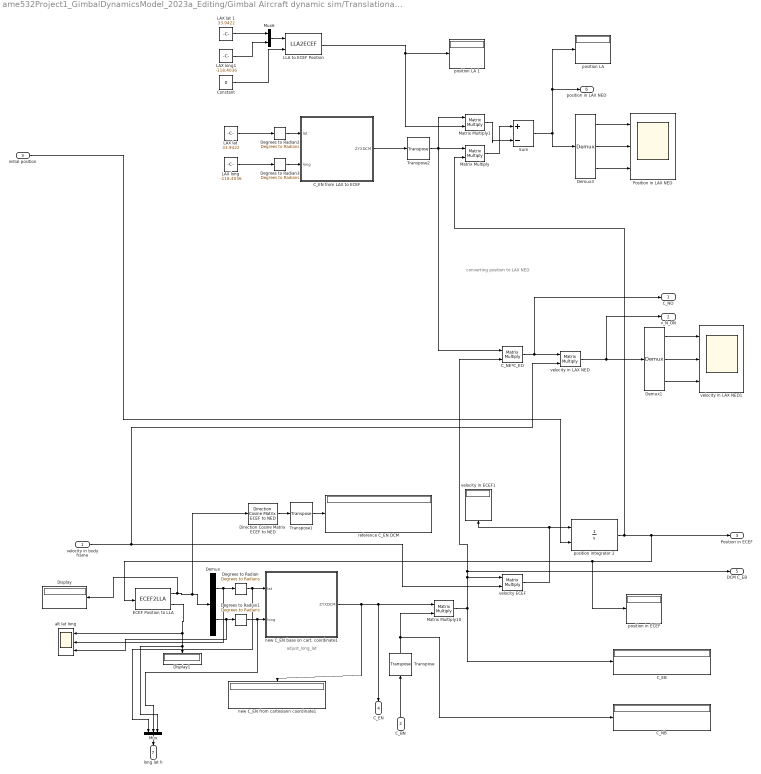
== system ame532Project1_GimbalDynamicsModel_2023a_Editing/Gimbal Aircraft dynamic sim/Translational Kinematics ==
  note: converting position to LAX NED
  note: adjust_long_lat
  velocity in body frame : Inport
  C_BN : Inport  Port=2
  initial position : Inport  Port=3
  C_EB : Display
  C_EN from LAX to ECEF : MATLAB Function  TreatAsAtomicUnit=on
  C_NB : Display
  C_NE*C_EO : Product  Multiplication=Matrix(*)
  Constant : Constant  Value=0
  Degrees to Radian{,1..3} (4 alike) : simulink_extras/Transformations/Degrees to Radians
  Demux : Demux  Outputs=2
  Demux1 : Demux  Outputs=3
  Demux3 : Demux  Outputs=3
  Direction Cosine Matrix ECEF to NED : aerolibtransform2/Direction Cosine Matrix ECEF to NED
  Display : Display
  Display1 : Display
  ECEF Position to LLA : ECEF2LLA  ptype=Custom  R=earthRadius
  "LAX lat " : Constant  Value=33.9422
  LAX lat 1 : Constant  Value=33.9422
  LAX long : Constant  Value=-118.4036
  LAX long1 : Constant  Value=-118.4036
  LLA to ECEF Position : LLA2ECEF  ptype=Custom  R=earthRadius
  Matrix Multiply : Product  Multiplication=Matrix(*)
  Matrix Multiply1 : Product  Multiplication=Matrix(*)
  Matrix Multiply10 : Product  Multiplication=Matrix(*)
  Mux : Mux  Inputs=3
  Mux6 : Mux  Inputs=2
  Position in LAX NED : Scope  NumInputPorts=3
  Sum : Sum  Inputs=|+-
  Transpose : matrix_library/Transpose
  Transpose1 : matrix_library/Transpose
  Transpose2 : matrix_library/Transpose
  alt lat long : Scope  NumInputPorts=3
  new C_EN base on cart. coordinate1 : MATLAB Function  TreatAsAtomicUnit=on
  new C_EN from cartesiann coordinate1 : Display
  "position LA " : Display
  position LA 1 : Display
  position in ECEF : Display
  position integrator 2 : Integrator  InitialConditionSource=external  InitialCondition=[6378100,0,0]'
  reference C_EN DCM : Display
  velocity ECEF : Product  Multiplication=Matrix(*)
  velocity in ECEF1 : Display
  velocity in LAX NED : Product  Multiplication=Matrix(*)
  velocity in LAX NED1 : Scope  NumInputPorts=3
  C_NO : Outport
  v_N_ON : Outport  Port=2
  Position in ECEF : Outport  Port=3
  C_EN : Outport  Port=4
  DCM C_EB : Outport  Port=5
  position in LAX NED : Outport  Port=6
  long lat h : Outport  Port=7
  wires:
  initial position/1 -> position integrator 2/2
  new C_EN base on cart. coordinate1/1(ZYXDCM) -> new C_EN from cartesiann coordinate1/1, C_EN/1, Matrix Multiply10/1
  Matrix Multiply10/1 -> C_EB/1, DCM C_EB/1, C_NE*C_EO/2, velocity ECEF/1
  velocity ECEF/1 -> position integrator 2/1, velocity in ECEF1/1
  velocity in body frame/1 -> velocity in LAX NED/2, velocity ECEF/2
  C_BN/1 -> Transpose/1
  ECEF Position to LLA/1 -> Direction Cosine Matrix ECEF to NED/1, Demux/1, Display/1
  ECEF Position to LLA/2 -> alt lat long/1, Mux/3, Display1/1
  Demux/1 -> Degrees to Radian/1, alt lat long/2
  Demux/2 -> alt lat long/3, Degrees to Radian1/1
  Degrees to Radian/1 -> Mux/1, new C_EN base on cart. coordinate1/1(lat)
  Degrees to Radian1/1 -> Mux/2, new C_EN base on cart. coordinate1/2(long)
  Transpose/1 -> C_NB/1, Matrix Multiply10/2
  Direction Cosine Matrix ECEF to NED/1 -> Transpose1/1
  Transpose1/1 -> reference C_EN DCM/1
  Mux/1 -> long lat h/1
  "LAX lat "/1 -> Degrees to Radian2/1
  LAX long/1 -> Degrees to Radian3/1
  Degrees to Radian2/1 -> C_EN from LAX to ECEF/1(lat)
  Degrees to Radian3/1 -> C_EN from LAX to ECEF/2(long)
  C_EN from LAX to ECEF/1(ZYXDCM) -> Transpose2/1
  Demux3/2 -> Position in LAX NED/2
  Demux3/3 -> Position in LAX NED/3
  Demux3/1 -> Position in LAX NED/1
  Transpose2/1 -> C_NE*C_EO/1, Matrix Multiply1/1, Matrix Multiply/1
  LAX long1/1 -> Mux6/2
  LAX lat 1/1 -> Mux6/1
  Constant/1 -> LLA to ECEF Position/2
  Mux6/1 -> LLA to ECEF Position/1
  LLA to ECEF Position/1 -> position LA 1/1, Matrix Multiply1/2
  Matrix Multiply/1 -> Sum/1
  Matrix Multiply1/1 -> Sum/2
  Sum/1 -> "position LA "/1, position in LAX NED/1, Demux3/1
  position integrator 2/1 -> Position in ECEF/1, ECEF Position to LLA/1, position in ECEF/1, Matrix Multiply/2
  C_NE*C_EO/1 -> C_NO/1, velocity in LAX NED/1
  Demux1/2 -> velocity in LAX NED1/2
  velocity in LAX NED/1 -> v_N_ON/1, Demux1/1
  Demux1/3 -> velocity in LAX NED1/3
  Demux1/1 -> velocity in LAX NED1/1

== system ame532Project1_GimbalDynamicsModel_2023a_Editing/Gimbal Aircraft dynamic sim/Unused tranlational kinmatics ==
  In1 : Inport
  In2 : Inport  Port=2
  In3 : Inport  Port=3
  C_EN4 : MATLAB Function  TreatAsAtomicUnit=on
  DCM4 : Display
  Matrix Multiply8 : Product  Multiplication=Matrix(*)
  Matrix Multiply9 : Product  Multiplication=Matrix(*)
  Scope7 : Scope
  Transpose : matrix_library/Transpose
  pitch4 : Constant  Value=pi/2
  position integrator 1 : Integrator  InitialConditionSource=external  InitialCondition=[6378100,0,0]'
  position vector2 : Display
  roll4 : Constant  Value=0
  velocity in earth frame : Display
  yaw4 : Constant  Value=0
  wires:
  Matrix Multiply9/1 -> DCM4/1, Matrix Multiply8/1
  position integrator 1/1 -> Scope7/1, position vector2/1
  C_EN4/1(ZYXDCM) -> Matrix Multiply9/1
  Matrix Multiply8/1 -> velocity in earth frame/1, position integrator 1/1
  yaw4/1 -> C_EN4/3(yaw)
  pitch4/1 -> C_EN4/2(pitch)
  Transpose/1 -> Matrix Multiply9/2
  roll4/1 -> C_EN4/1(roll)
  In2/1 -> Matrix Multiply8/2
  In1/1 -> position integrator 1/2
  In3/1 -> Transpose/1

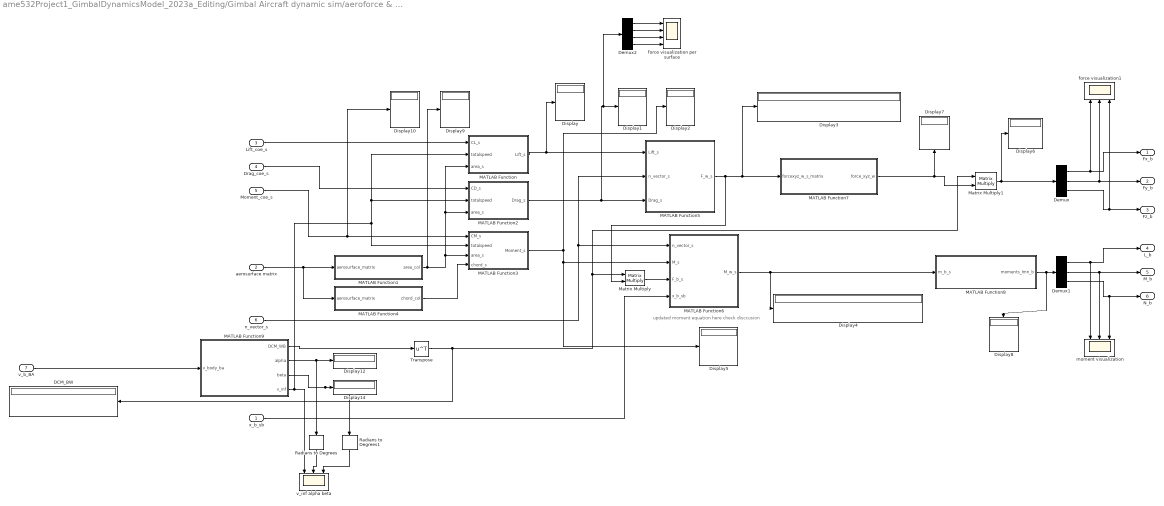
== system ame532Project1_GimbalDynamicsModel_2023a_Editing/Gimbal Aircraft dynamic sim/aeroforce & moment block ==
  note: updated moment equation here check disccusion
  x_b_sb : Inport
  aerosurface matrix : Inport  Port=2
  Lift_coe_s : Inport  Port=3
  Drag_coe_s : Inport  Port=4
  Moment_coe_s : Inport  Port=5
  n_vector_s : Inport  Port=6
  v_b_BA : Inport  Port=7
  DCM_BW : Display
  Demux : Demux  Outputs=3
  Demux1 : Demux  Outputs=3
  Demux2 : Demux
  Display{,1..10,12,14} (13 alike) : Display
  MATLAB Function : MATLAB Function  TreatAsAtomicUnit=on
  MATLAB Function1 : MATLAB Function  TreatAsAtomicUnit=on
  MATLAB Function2 : MATLAB Function  TreatAsAtomicUnit=on
  MATLAB Function3 : MATLAB Function  TreatAsAtomicUnit=on
  MATLAB Function4 : MATLAB Function  TreatAsAtomicUnit=on
  MATLAB Function5 : MATLAB Function  TreatAsAtomicUnit=on
  MATLAB Function6 : MATLAB Function  TreatAsAtomicUnit=on
  MATLAB Function7 : MATLAB Function  TreatAsAtomicUnit=on
  MATLAB Function8 : MATLAB Function  TreatAsAtomicUnit=on
  MATLAB Function9 : MATLAB Function  TreatAsAtomicUnit=on
  Matrix Multiply : Product  Multiplication=Matrix(*)
  Matrix Multiply1 : Product  Multiplication=Matrix(*)
  Radians to Degrees : simulink_extras/Transformations/Radians to Degrees
  Radians to Degrees1 : simulink_extras/Transformations/Radians to Degrees
  Transpose : Math  Operator=transpose
  force visualization per surface : Scope  NumInputPorts=4
  force visualization1 : Scope  NumInputPorts=3
  moment visualization : Scope  NumInputPorts=3
  v_inf alpha beta : Scope  NumInputPorts=3
  Fx_b : Outport
  Fy_b : Outport  Port=2
  Fz_b : Outport  Port=3
  L_b : Outport  Port=4
  M_b : Outport  Port=5
  N_b : Outport  Port=6
  wires:
  Lift_coe_s/1 -> MATLAB Function/1(CL_s)
  MATLAB Function9/4(v_inf) -> v_inf alpha beta/1, MATLAB Function2/2(totalspeed), MATLAB Function/2(totalspeed), MATLAB Function3/2(totalspeed)
  aerosurface matrix/1 -> MATLAB Function4/1(aerosurface_matrix), MATLAB Function1/1(aerosurface_matrix)
  MATLAB Function1/1(area_col) -> Display9/1, MATLAB Function2/3(area_s), MATLAB Function/3(area_s), MATLAB Function3/3(area_s)
  Drag_coe_s/1 -> MATLAB Function2/1(CD_s)
  Moment_coe_s/1 -> Display10/1, MATLAB Function3/1(CM_s)
  MATLAB Function4/1(chord_col) -> MATLAB Function3/4(chord_s)
  n_vector_s/1 -> MATLAB Function5/2(n_vector_s), MATLAB Function6/1(n_vector_s)
  MATLAB Function/1(Lift_s) -> Display/1, MATLAB Function5/1(Lift_s)
  MATLAB Function2/1(Drag_s) -> MATLAB Function5/3(Drag_s), Demux2/1, Display1/1
  MATLAB Function3/1(Moment_s) -> Display5/1, MATLAB Function6/2(M_s), Display2/1
  MATLAB Function6/1(M_w_s) -> Display4/1, MATLAB Function8/1(m_b_s)
  Matrix Multiply/1 -> MATLAB Function6/3(F_b_s)
  x_b_sb/1 -> MATLAB Function6/4(x_b_sb)
  MATLAB Function5/1(F_w_s) -> Matrix Multiply/2, Display3/1, MATLAB Function7/1(forcexyz_w_s_matrix)
  MATLAB Function7/1(force_xyz_w) -> Matrix Multiply1/2, Display7/1
  MATLAB Function8/1(moments_lmn_b) -> Demux1/1, Display8/1
  Matrix Multiply1/1 -> Demux/1, Display6/1
  MATLAB Function9/1(DCM_WB) -> Transpose/1
  v_b_BA/1 -> MATLAB Function9/1(v_body_ba)
  MATLAB Function9/2(alpha) -> Radians to Degrees/1, Display12/1
  MATLAB Function9/3(beta) -> Display14/1, Radians to Degrees1/1
  Demux1/1 -> L_b/1, moment visualization/1
  Demux1/2 -> M_b/1, moment visualization/2
  Demux1/3 -> moment visualization/3, N_b/1
  Demux/1 -> Fx_b/1, force visualization1/1
  Demux/2 -> Fy_b/1, force visualization1/2
  Demux/3 -> Fz_b/1, force visualization1/3
  Transpose/1 -> Matrix Multiply1/1, Matrix Multiply/1, DCM_BW/1
  Radians to Degrees/1 -> v_inf alpha beta/2
  Radians to Degrees1/1 -> v_inf alpha beta/3
  Demux2/4 -> force visualization per surface/4
  Demux2/3 -> force visualization per surface/3
  Demux2/2 -> force visualization per surface/2
  Demux2/1 -> force visualization per surface/1
